simulink model "SimulinkModel_FINAL"  (R2023b)
settings: Solver=VariableStepAuto  StartTime=0.0  StopTime=5  RelTol=1e-3
libraries: simulink x2, dspvision x2, commcnvcod2 x2, commchan3 x2, commdigbbndpm3 x2, commfilt2 x2, commsink2 x1, dspindex x1
settings Model: Creator=user  LastModifiedBy=sidha

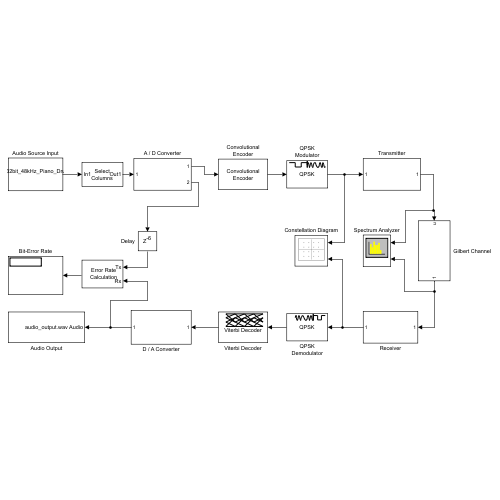
[thumbnail: Simulink's stored preview of the top-level diagram]
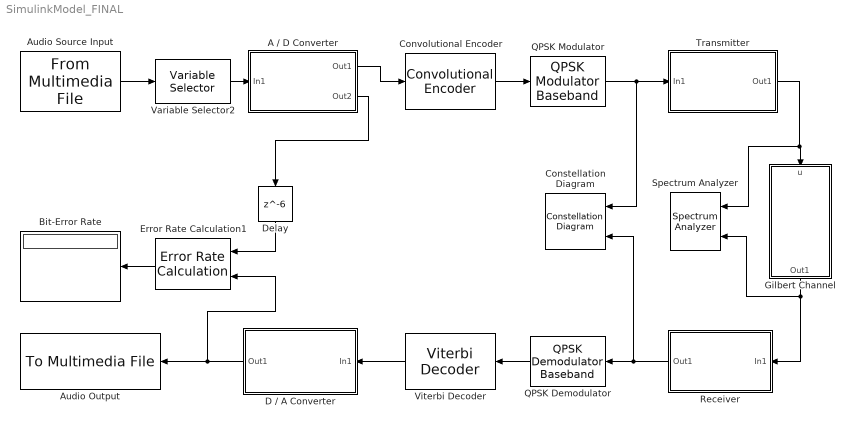
== system SimulinkModel_FINAL ==
  A / D Converter : Subsystem
  Audio Output : dspvision/To Multimedia File  outputFilename=C:\Users\sidha\OneDrive\Documents\MATLAB\ELEC391_Sound_Files\audio_output.wav  streamSelection=Audio only  videoCompressor=None (uncompressed)  audioCompressor=None (uncompressed)  imagePorts=One multidimensional signal  fileType=WAV  audioDatatype=16-bit integer  fourcc=RGB  videoQuality=75  mj2000CompFactor=10
      settings: LibrarySourceBlock=dspsnks4/To Multimedia File
  Audio Source Input : dspvision/From Multimedia File  inputFilename=C:\Users\sidha\OneDrive\Documents\MATLAB\ELEC391_Sound_Files\Stereo_32bit_48kHz_Piano_Drums.wav  readRange=[1 Inf]  loop=on  numPlays=1  outputStreams=Audio only  videoDataType=single  audioDataType=int16  inheritSampleTime=on  userDefinedSampleTime=1/30  noAudioOutput=off  isIntensityVideo=off  fourcc=RGB  colorVideoFormat=Separate color signals  outputEOF=off  dataOrg=Column-major  audioFrameSize=1  computeAudioFrameSize=off  outSamplingMode=Sample based
      settings: LibrarySourceBlock=dspsrcs4/From Multimedia File
  Bit-Error Rate : Display
  Constellation Diagram : ConstellationDiagram  NumInputPorts=2  WindowPosition=[-97.000000,0.000000,1536.000000,793.000000,]  Visible=on  ScopeFrameLocation=window  ReferenceConstellation="{[0.7071+0.7071i          -0.7071+0.7071i          -0.7071-0.7071i            0.707-0.7071i][0.7071+0.7071i          -0.7071+0.7071i          -0.7071-0.7071i            0.707-0.7071i]}"  XLimits=[-1.46,1.46]  YLimits=[-1.38,1.38]  ShowLegend=on
  Convolutional Encoder : commcnvcod2/Convolutional Encoder  trellis=poly2trellis(7, [171 133])  opMode=Continuous  DelayedResetAction=off  hasIniStPort=off  hasFinStPort=off  usePuncVector=off  punctureVector=[1; 1; 0; 1; 0; 1]  reset=Unused parameter value
  D / A Converter : Subsystem
  Delay : Delay  DelayLength=6
  Error Rate Calculation1 : commsink2/Error Rate Calculation  N=0  st_delay=6  cp_mode=Entire frame  subframe=[]  PMode=Port  WsName=ErrorVec  RsMode2=off  stop=off  numErr=100  maxBits=1e6
      settings: LibrarySourceBlock=|
      | commhdlsink/Error Rate
      | Calculation
  Gilbert Channel : Subsystem
  QPSK Demodulator : commdigbbndpm3/QPSK Demodulator Baseband  OutType=Bit  DecType=Hard decision  VarSource=Dialog  Variance=1  Dec=Gray  Ph=pi/4  outDtype1=Inherit via internal rule  outDtype2=Inherit via internal rule  derotateFactorWordLen=16  derotateFactorDataTypeStr=Inherit: Same word length as input  derotateFactorLastDataTypeStr=Inherit: Same word length as input
  QPSK Modulator : commdigbbndpm3/QPSK Modulator Baseband  InType=Bit  Enc=Gray  Ph=pi/4  outDtype=double  outWordLen=16  outUDDataType=sfix(16)  outFracLenMode=Best precision  outFracLen=15  outDataTypeStr=double  outLastDataTypeStr=double
  Receiver : Subsystem
  Spectrum Analyzer : SpectrumAnalyzer  NumInputPorts=2  WindowPosition=[-5.000000,120.000000,1264.000000,633.000000,]  Visible=on  ScopeFrameLocation=window  SampleRate=44.1e3  PlotAsTwoSidedSpectrum=off  FrequencySpan=Start and stop frequencies  StartFrequency=0  StopFrequency=300000  YLimits=[-127.2409805,16.90943263]
  Transmitter : Subsystem
  Variable Selector2 : dspindex/Variable Selector  NumInputs=1  rowsOrCols=Columns  IdxMode=Fixed  Elements=[1]  ZerOneIdxMode=One-based  errmode=Clip Index  FillMode=off  FillValues=0
  Viterbi Decoder : commcnvcod2/Viterbi Decoder  trellis=poly2trellis(7, [171 133])  isPunctured=off  punctureVector=[1; 1; 0; 1; 0; 1]  erasures=off  dectype=Hard decision  nsdecb=4  runSigValErrCheck=off  tbdepth=32  opmode=Continuous  reset=off  delayedResetAction=off  smWordLength=16  outDataType=Inherit via internal rule
  wires:
  Viterbi Decoder/1 -> D / A Converter/1(In1)
  D / A Converter/1(Out1) -> Audio Output/1, Error Rate Calculation1/2
  Delay/1 -> Error Rate Calculation1/1
  QPSK Modulator/1 -> Constellation Diagram/1, Transmitter/1(In1)
  Audio Source Input/1 -> Variable Selector2/1
  Error Rate Calculation1/1 -> Bit-Error Rate/1
  Transmitter/1(Out1) -> Gilbert Channel/1(u), Spectrum Analyzer/1
  Gilbert Channel/1(Out1) -> Spectrum Analyzer/2, Receiver/1(In1)
  Convolutional Encoder/1 -> QPSK Modulator/1
  QPSK Demodulator/1 -> Viterbi Decoder/1
  Receiver/1(Out1) -> QPSK Demodulator/1, Constellation Diagram/2
  Variable Selector2/1 -> A / D Converter/1(In1)
  A / D Converter/1(Out1) -> Convolutional Encoder/1
  A / D Converter/2(Out2) -> Delay/1

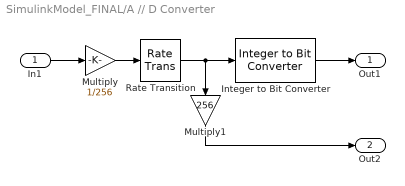
== system SimulinkModel_FINAL/A // D Converter ==
  In1 : Inport
  Integer to Bit Converter : simulink/Logic and Bit Operations/Integer to Bit Converter  nbits=8  signedInputValues=Signed  bitOrder=MSB first  outDtype=boolean
      settings: LibrarySourceBlock=|
      | commutil2/Integer to Bit
      | Converter
  Multiply : Gain  Gain=1/256  OutDataTypeStr=int16  RndMeth=Zero
  Multiply1 : Gain  Gain=256  OutDataTypeStr=int16
  Rate Transition : RateTransition  Integrity=off  Deterministic=off  OutPortSampleTime=1/20000
  Out1 : Outport
  Out2 : Outport  Port=2
  wires:
  Multiply1/1 -> Out2/1
  Rate Transition/1 -> Integer to Bit Converter/1, Multiply1/1
  Multiply/1 -> Rate Transition/1
  Integer to Bit Converter/1 -> Out1/1
  In1/1 -> Multiply/1

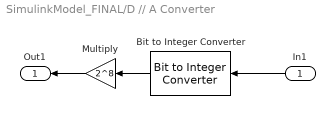
== system SimulinkModel_FINAL/D // A Converter ==
  In1 : Inport
  Bit to Integer Converter : simulink/Logic and Bit Operations/Bit to Integer Converter  nbits=8  bitOrder=MSB first  signedOutputValues=Signed  outDtype=Inherit via internal rule  outDtypeSigned=int16
      settings: LibrarySourceBlock=|
      | commutil2/Bit to Integer
      | Converter
  Multiply : Gain  Gain=2^8  OutDataTypeStr=int16
  Out1 : Outport
  wires:
  In1/1 -> Bit to Integer Converter/1
  Bit to Integer Converter/1 -> Multiply/1
  Multiply/1 -> Out1/1

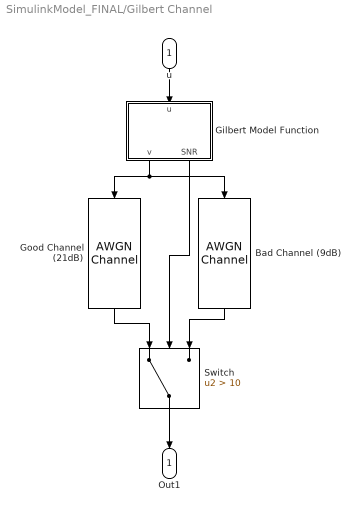
== system SimulinkModel_FINAL/Gilbert Channel ==
  u : Inport
  Bad Channel (9dB) : commchan3/AWGN Channel  LegacyMode=off  NoiseMethod="Signal to noise ratio  (SNR)"  noiseMode="Signal to noise ratio  (SNR)"  EbNo=10  EsNo=100  SNR=9  BitsPerSymbol=1  SignalPower=1  SamplesPerSymbol=4  SymbolPeriod=1  VarianceSource=Parameter  Variance=1  RandomStream=Global stream  Seed=67  SimulateUsing=Code generation
  Gilbert Model Function : MATLAB Function  TreatAsAtomicUnit=on
  Good Channel (21dB) : commchan3/AWGN Channel  LegacyMode=off  NoiseMethod="Signal to noise ratio  (SNR)"  noiseMode="Signal to noise ratio  (SNR)"  EbNo=10  EsNo=100  SNR=21  BitsPerSymbol=1  SignalPower=1  SamplesPerSymbol=4  SymbolPeriod=1  VarianceSource=Parameter  Variance=1  RandomStream=Global stream  Seed=67  SimulateUsing=Code generation
  Switch : Switch  Criteria=u2 > Threshold  Threshold=10  SaturateOnIntegerOverflow=off  InputSameDT=off
  Out1 : Outport
  wires:
  u/1 -> Gilbert Model Function/1(u)
  Gilbert Model Function/1(v) -> Bad Channel (9dB)/1, Good Channel (21dB)/1
  Gilbert Model Function/2(SNR) -> Switch/2
  Switch/1 -> Out1/1
  Bad Channel (9dB)/1 -> Switch/3
  Good Channel (21dB)/1 -> Switch/1

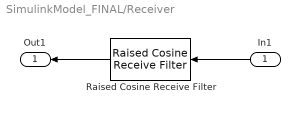
== system SimulinkModel_FINAL/Receiver ==
  In1 : Inport
  Raised Cosine Receive Filter : commfilt2/Raised Cosine Receive Filter  filtType=Normal  R=0.25  filtSpan=16  N=6  downFactor=6  downOffset=0  filterGain=1  InputProcessing=Columns as channels (frame based)  RateOptions=Enforce single-rate processing  framing=Mute  checkCoeff=on  variableName=rcRxFilt  currentFiltSpan=10  D=5  inputOffset=0  sampMode=Mute  saveAsFlag=0  rateMode=Downsampling  checkGain=Normalized  launchFVT=on  roundingMode=Floor  overflowMode=off  coeffDataTypeStr=Inherit: Same word length as input  coeffMin=[]  coeffMax=[]  coeffLastDataTypeStr=Inherit: Same word length as input  accumDataTypeStr=Inherit: Same as product output  accumLastDataTypeStr=Inherit: Same as product output  outputDataTypeStr=Inherit: Same as accumulator  outputMin=[]  outputMax=[]  outputLastDataTypeStr=Inherit: Same as accumulator
  Out1 : Outport
  wires:
  In1/1 -> Raised Cosine Receive Filter/1
  Raised Cosine Receive Filter/1 -> Out1/1

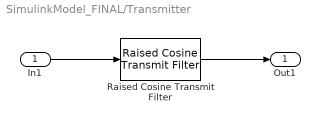
== system SimulinkModel_FINAL/Transmitter ==
  In1 : Inport
  Raised Cosine Transmit Filter : commfilt2/Raised Cosine Transmit Filter  filtType=Normal  R=0.25  filtSpan=16  N=6  filterGain=1  InputProcessing=Columns as channels (frame based)  RateOptions=Enforce single-rate processing  framing=Mute  checkCoeff=on  variableName=rcTxFilt  checkGain=Normalized  sampMode=Mute  saveAsFlag=0  currentFiltSpan=10  D=(10)/2  launchFVT=on  roundingMode=Floor  overflowMode=off  coeffDataTypeStr=Inherit: Same word length as input  coeffMin=[]  coeffMax=[]  coeffLastDataTypeStr=Inherit: Same word length as input  outputDataTypeStr=Inherit: Same as accumulator  outputMin=[]  outputMax=[]  outputLastDataTypeStr=Inherit: Same as accumulator
  Out1 : Outport
  wires:
  In1/1 -> Raised Cosine Transmit Filter/1
  Raised Cosine Transmit Filter/1 -> Out1/1

== matlab function SimulinkModel_FINAL/Gilbert Channel/Gilbert Model Function ==
  data: v output; u input; SNR output
function [v, SNR] = gilbert(u)

% Define Transition Matrix
P = [0.95, 0.05; 0.2, 0.8];

% Persistent variable to hold the current state
persistent presentstate;

% Initialize the state if it is the first run
if isempty(presentstate)
    presentstate = 1; % Start in state 1 (Good)
    SNR = 21;
end

% Determine the next state based on the current state and input
if presentstate == 1
    if rand < P(1,2)
        nextstate = 2; % Transition to bad state
    else
        nextstate = 1; % Remain in good state
    end
else
    if rand < P(2,1)
        nextstate = 1; % Transition to good state
    else
        nextstate = 2; % Remain in bad state
    end
end

% Update the present state
presentstate = nextstate;

% Set the SNR value based on the current state
if presentstate == 1
    SNR = 21; % Good state
else
    SNR = 10; % Bad state
end

v = u;
